simulink model "acDynModelGolfTenueModaleBAD"  (R2019a)
settings: Solver=VariableStepAuto  StartTime=0.0  StopTime=10  RelTol=1e-3
values from neighbouring files (symbols this model uses):
  dPHRTrim = trimVal(1)    [mainProjetCADV_2a.m]
  dthrIdle = 0.1    [mainProjetCADV_2a.m]
  hTrim = hTrimFL*FL2M    [mainProjetCADV_2a.m]
  km = trim.kmass(choix)    [utGetTrimPoint.m]
  KTS2MS = 1852 / 3600    (= 0.514444444444)    [mainProjetCADV_2a.m]    (also in utAcDynamicsFunction.m)
  ms = trim.mStat(choix)    [utGetTrimPoint.m]
  VaTrim = utEas2Tas(Eas_KTS*KTS2MS, hTrimFL*FL2M)    [mainProjetCADV_2a.m]
  xTrim = zeros(TOTAL_SV, 1)    [mainProjetCADV_2a.m]
undefined symbols (not defined in the file or in its folder): aircraftChosen, Ctas, Eas_KTS, K5, K6, Kd, Ki, Kp, MS2KTS
settings Model: Creator=bourdiul  LastModifiedBy=ulyss

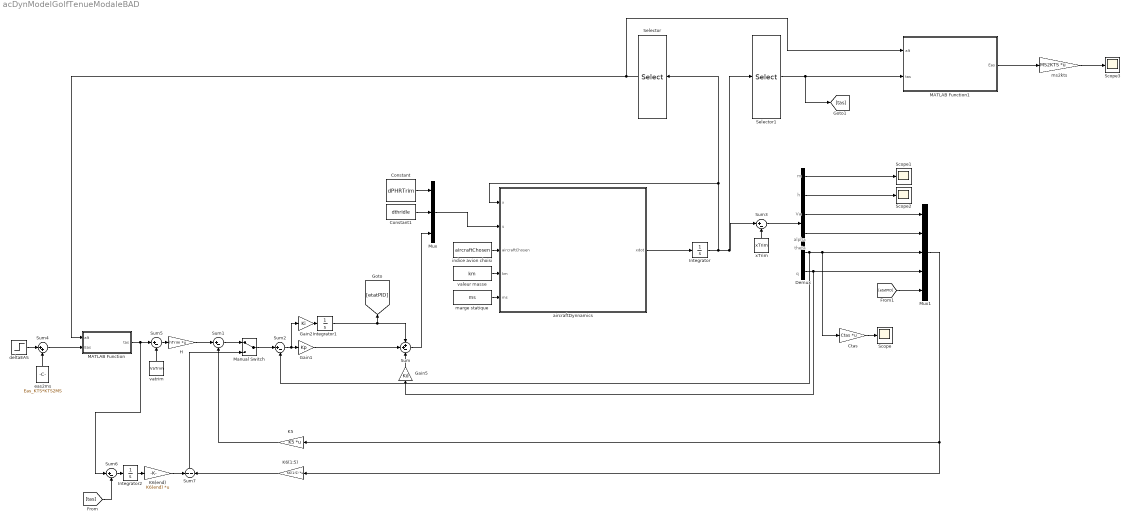
== system acDynModelGolfTenueModaleBAD ==
  note: m
  note: h
  note: Va
  note: alpha
  note: theta
  note: q
  Constant : Constant  Value=dPHRTrim
  Constant1 : Constant  Value=dthrIdle
  Ctas : Gain  Gain=Ctas  Multiplication=Matrix(K*u) (u vector)
  Demux : Demux  Outputs=6
  Gain1 : Gain  Gain=Kp
  Gain2 : Gain  Gain=Ki
  Gain5 : Gain  Gain=Kd
  H : Gain  Gain=hTrim  Multiplication=Matrix(K*u) (u vector)
  Integrator : Integrator  InitialCondition=xTrim
  Integrator1 : Integrator
  Integrator2 : Integrator
  K5 : Gain  Gain=K5  Multiplication=Matrix(K*u) (u vector)
  K6(1:5) : Gain  Gain=K6(1:5)  Multiplication=Matrix(K*u) (u vector)
  K6(end) : Gain  Gain=K6(end)  Multiplication=Matrix(K*u) (u vector)
  MATLAB Function : MATLAB Function  TreatAsAtomicUnit=on
  MATLAB Function1 : MATLAB Function  TreatAsAtomicUnit=on
  Manual Switch : ManualSwitch
  Mux : Mux  Inputs=3
  Mux1 : Mux  Inputs=5
  Scope{,1..3} (4 alike) : Scope
  Selector : Selector  IndexMode=Zero-based  InputPortWidth=6  IndexOptions=Index vector (dialog)  Indices=1  OutputSizes=1
  Selector1 : Selector  InputPortWidth=6  IndexOptions=Index vector (dialog)  Indices=3  OutputSizes=1
  Sum : Sum  Inputs=++-
  Sum{1..3,5..6} (5 alike) : Sum  Inputs=|+-
  Sum4 : Sum  Inputs=|++
  Sum7 : Sum  Inputs=-|-
  aircraftDynnamics : MATLAB Function  TreatAsAtomicUnit=on
  deltaEAS : Step  Time=0  After=5  SampleTime=0
  eas2ms : Constant  Value=Eas_KTS*KTS2MS
  indice avion choisi : Constant  Value=aircraftChosen
  marge statique : Constant  Value=ms
  ms2kts : Gain  Gain=MS2KTS  Multiplication=Matrix(K*u) (u vector)
  valeur masse : Constant  Value=km
  vatrim : Constant  Value=VaTrim
  xTrim : Constant  Value=xTrim
  wires:
  marge statique/1 -> aircraftDynnamics/5(ms)
  Integrator/1 -> Selector1/1, Sum3/1, Selector/1, aircraftDynnamics/1(x)
  Demux/6 -> Gain5/1, Mux1/4
  Mux/1 -> aircraftDynnamics/2(u)
  Demux/2 -> Scope2/1
  indice avion choisi/1 -> aircraftDynnamics/3(aircraftChosen)
  Demux/3 -> Mux1/1
  valeur masse/1 -> aircraftDynnamics/4(km)
  aircraftDynnamics/1(xdot) -> Integrator/1
  Demux/4 -> Mux1/2
  Constant1/1 -> Mux/2
  Constant/1 -> Mux/1
  Demux/1 -> Scope1/1
  Gain5/1 -> Sum/3
  deltaEAS/1 -> Sum4/1
  Gain1/1 -> Sum/2
  Integrator1/1 -> [etatPID], Sum/1
  Gain2/1 -> Integrator1/1
  Sum2/1 -> Gain2/1, Gain1/1
  Sum/1 -> Mux/3
  Manual Switch/1 -> Sum2/1
  Sum1/1 -> Manual Switch/1
  H/1 -> Sum1/1
  Sum5/1 -> H/1
  vatrim/1 -> Sum5/2
  MATLAB Function/1(tas) -> Sum6/1, Sum5/1
  eas2ms/1 -> Sum4/2
  Sum4/1 -> MATLAB Function/2(Eas)
  Selector/1 -> MATLAB Function1/1(alt), MATLAB Function/1(alt)
  Selector1/1 -> [tas], MATLAB Function1/2(tas)
  MATLAB Function1/1(Eas) -> ms2kts/1
  ms2kts/1 -> Scope3/1
  [tas] -> Sum6/2
  Sum6/1 -> Integrator2/1
  Integrator2/1 -> K6(end)/1
  K6(1:5)/1 -> Sum7/2
  K6(end)/1 -> Sum7/1
  Sum7/1 -> Manual Switch/2
  K5/1 -> Sum1/2
  Mux1/1 -> K6(1:5)/1, K5/1
  xTrim/1 -> Sum3/2
  Sum3/1 -> Demux/1
  [etatPID] -> Mux1/5
  Ctas/1 -> Scope/1
  Demux/5 -> Ctas/1, Mux1/3, Sum2/2

== matlab function acDynModelGolfTenueModaleBAD/MATLAB Function ==
  data: alt input; Eas input; tas output
function tas = utEas2tas(alt, Eas)
    %tas, Eas (%equivalent vitesse) en m/s
    %alt en m
    %cf. http://www.hochwarth.com/misc/AviationCalculator.html
    tas = sqrt(utRho(0)/utRho(alt))*Eas;
end

== matlab function acDynModelGolfTenueModaleBAD/aircraftDynnamics ==
  data: x input; u input; xdot output; aircraftChosen input; km input; ms input
function xdot = aircraftDynamics(x,u, aircraftChosen,km,ms)
    TOTAL_SV = 6;
    xIn = zeros(TOTAL_SV,1);
    xIn = x;
    
	TOTAL_CMD = 3;
    uIn = zeros(TOTAL_CMD,1);
    uIn = u;
    
    xdot = utAcDynamicsFunction(xIn,uIn, aircraftChosen,km,ms);
end %aircraftDynamics

== matlab function acDynModelGolfTenueModaleBAD/MATLAB Function1 ==
  data: alt input; tas input; Eas output
function Eas = utTas2Eas(alt, tas)
    %tas, Eas(%equivalent vitesse) en m/s
    %alt en m
    %cf. http://www.hochwarth.com/misc/AviationCalculator.html
    Eas = sqrt(utRho(alt)/utRho(0))*tas;
end
